simulink model "Tone"  (R2017b)
settings: Solver=VariableStepAuto  StartTime=0.0  StopTime=inf  RelTol=1e-3
undefined symbols (not defined in the file): serial
libraries: instrumentlib x2, dspsnks4 x1
settings Model: Creator=pipe  LastModifiedBy=pipe

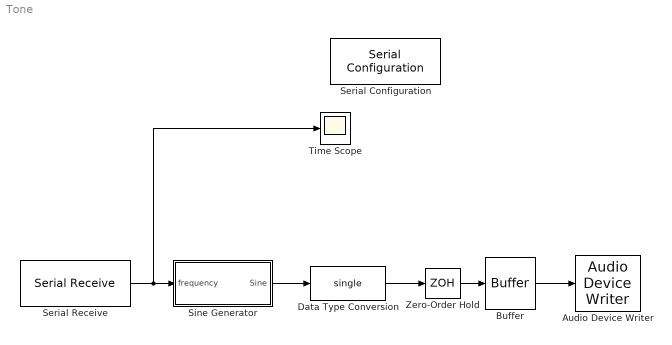
== system Tone ==
  Audio Device Writer : dspsnks4/Audio Device Writer  Driver=DirectSound  Device=Default  InheritSampleRate=on  SampleRate=40000  BitDepth=16-bit integer  BufferSize=4096  NumBuffers=10  DefaultOutputChannelMapping=on  OutputChannelMapping=1:2  OutputNumUnderrunSamples=off  DriverIdx=1  DeviceWarnFlag=''
  Buffer : Buffer  N=16  OutputFrames=off
  Data Type Conversion : DataTypeConversion  OutDataTypeStr=single
  Serial Configuration : instrumentlib/Serial Configuration  Priority=-200000  ComPortMenu=COM7  ComPort=COM7  ObjConstructor=serial('COM7');  BaudRate=115200  DataBits=8  Parity=none  StopBits=1  FlowControl=none  Timeout=10  ByteOrder=LittleEndian
  Serial Receive : instrumentlib/Serial Receive  ComPortMenu=COM7  ComPort=COM7  ObjConstructor=serial('COM7');  Header=~  Terminator=0  DataSize=[1 1]  DataType=uint32  EnableBlockingMode=on  ActionDataUnavailable=Output last received value  CustomValue=0  SampleTime=0.01
  Sine Generator : Subsystem  TreatAsAtomicUnit=on
  Time Scope : Scope
  Zero-Order Hold : ZeroOrderHold  SampleTime=3/11520
  wires:
  Buffer/1 -> Audio Device Writer/1
  Data Type Conversion/1 -> Zero-Order Hold/1
  Zero-Order Hold/1 -> Buffer/1
  Serial Receive/1 -> Time Scope/1, Sine Generator/1("frequency ")
  Sine Generator/1(Sine) -> Data Type Conversion/1

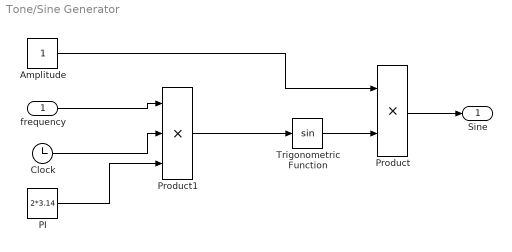
== system Tone/Sine Generator ==
  "frequency " : Inport
  "Amplitude " : Constant
  Clock : Clock
  "PI " : Constant  Value=2*3.14
  Product : Product
  Product1 : Product  Inputs=3
  Trigonometric Function : Trigonometry
  Sine : Outport
  wires:
  Product/1 -> Sine/1
  Clock/1 -> Product1/2
  "Amplitude "/1 -> Product/1
  Trigonometric Function/1 -> Product/2
  "frequency "/1 -> Product1/1
  Product1/1 -> Trigonometric Function/1
  "PI "/1 -> Product1/3
